simulink model "obstacleAvoidanceUsingOpticalFlow"  (R2021a)
settings: Solver=VariableStepAuto  StartTime=0.0  StopTime=30  RelTol=1e-3
PostLoadFcn:
  | %Add subfolders to path
  | addpath('virtualworld');
InitFcn:
  | startScript;
values from neighbouring files (symbols this model uses):
  angularVelocity = [0 0 -0.01]    [startScript.m]
  angularVelocityforLanding = [0 0 0.01]    [startScript.m]
  delta = 0.1    [startScript.m]
  dronestartlocation = [-1.5 0 4]    [startScript.m]
  finalHoverHeight = 0.8    [startScript.m]
  helipadLocation = [14 0.29 4]    [startScript.m]
  linearVelocity = [0.6 0.05 .2]    [startScript.m]
  switchingXLimit = 12.0    (= 12)    [startScript.m]
undefined symbols (not defined in the file or in its folder): gcbh, Horn, Rec, Schunck, SDTV, vrmfunc
libraries: vrlib x6, pid_lib x4, sharedtransform x2, visionconversions x1, visiontextngfix x1, visionanalysis x1
settings Model: Creator=91967  LastModifiedBy=mmordeka
settings SolverCC: AlgebraicLoopSolver=TrustRegion
settings DebuggingCC: SFMachineParentedDataDiag=warning

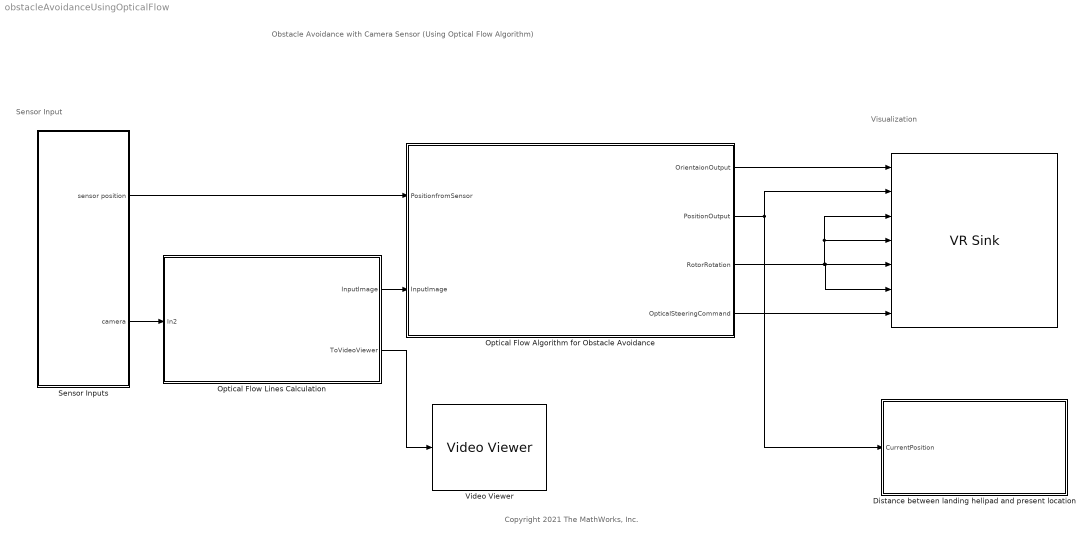
== system obstacleAvoidanceUsingOpticalFlow ==
  note: Sensor Input
  note: Copyright 2021 The MathWorks, Inc.
  note: Obstacle Avoidance with Camera Sensor
      | (Using Optical Flow Algorithm)
  note: Visualization
  "    " : vrlib/VR Sink  InstantiateOnLoad=on  SampleTime=0.04  ViewEnable=on  RemoteChange=off  RemoteView=off  FieldsWritten=UAV.rotation.4.1.1.double#UAV.translation.3.1.1.double#UAV_Body.Propeller_Mode_1.1.1.1.double#UAV_Body.Propeller_Mode_2.1.1.1.double#UAV_Body.Propeller_Mode_3.1.1.1.double#UAV_Body.Propeller_Mode_4.1.1.1.double#HUDText1.string.1.-1.1.char  WorldFileName=slv3.x3d  WorldDescription=Obstacle Avoidance with Camera Sensor (Using Optical Flow Algorithm)  AutoView=off  VideoDimensions=[]  AllowVariableSize=off
  " Distance between landing helipad and present location" : Subsystem
  " Optical Flow Algorithm for Obstacle Avoidance" : Subsystem
  Optical Flow Lines Calculation : Subsystem
  Sensor Inputs : Subsystem
  Video Viewer : VideoViewer  FigPos=[1242 576 441 340]  OpenAtMdlStart=off
  wires:
  " Optical Flow Algorithm for Obstacle Avoidance"/2(PositionOutput) -> " Distance between landing helipad and present location"/1(CurrentPosition), "    "/2
  Optical Flow Lines Calculation/1(InputImage) -> " Optical Flow Algorithm for Obstacle Avoidance"/2(InputImage)
  Optical Flow Lines Calculation/2(ToVideoViewer) -> Video Viewer/1
  Sensor Inputs/1(sensor position) -> " Optical Flow Algorithm for Obstacle Avoidance"/1(PositionfromSensor)
  Sensor Inputs/2(camera) -> Optical Flow Lines Calculation/1(In2)
  " Optical Flow Algorithm for Obstacle Avoidance"/1(OrientaionOutput) -> "    "/1
  " Optical Flow Algorithm for Obstacle Avoidance"/3(RotorRotation) -> "    "/4, "    "/3, "    "/6, "    "/5
  " Optical Flow Algorithm for Obstacle Avoidance"/4(OpticalSteeringCommand) -> "    "/7

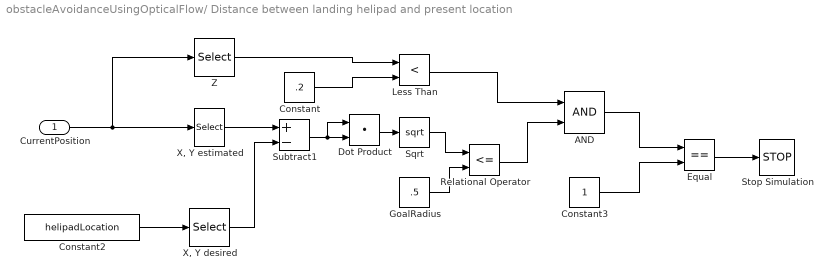
== system obstacleAvoidanceUsingOpticalFlow/ Distance between landing helipad and present location ==
  CurrentPosition : Inport
  AND : Logic  IconShape=distinctive  AllPortsSameDT=off  OutDataTypeStr=boolean
  Constant : Constant  Value=.2
  Constant2 : Constant  Value=helipadLocation
  Constant3 : Constant
  Dot Product : DotProduct  InputSameDT=on  OutDataTypeStr=Inherit: Inherit via internal rule
  Equal : RelationalOperator  Operator===  OutDataTypeStr=boolean  RndMeth=Simplest
  GoalRadius : Constant  Value=.5
  Less Than : RelationalOperator  Operator=<  OutDataTypeStr=boolean  RndMeth=Simplest
  Relational Operator : RelationalOperator  Operator=<=  OutDataTypeStr=boolean  RndMeth=Simplest
  Sqrt : Sqrt  SaturateOnIntegerOverflow=on
  Stop Simulation : Stop
  Subtract1 : Sum  Inputs=+-
  "X, Y desired" : Selector  InputPortWidth=3  IndexOptions=Index vector (dialog)  Indices=[1 3]  OutputSizes=1
  "X, Y estimated" : Selector  InputPortWidth=3  IndexOptions=Index vector (dialog)  Indices=[1 3]  OutputSizes=1
  Z : Selector  InputPortWidth=3  IndexOptions=Index vector (dialog)  Indices=[2]  OutputSizes=1
  wires:
  GoalRadius/1 -> Relational Operator/2
  Subtract1/1 -> Dot Product/1, Dot Product/2
  Dot Product/1 -> Sqrt/1
  Sqrt/1 -> Relational Operator/1
  "X, Y estimated"/1 -> Subtract1/1
  CurrentPosition/1 -> Z/1, "X, Y estimated"/1
  "X, Y desired"/1 -> Subtract1/2
  Constant3/1 -> Equal/2
  Equal/1 -> Stop Simulation/1
  Constant2/1 -> "X, Y desired"/1
  AND/1 -> Equal/1
  Relational Operator/1 -> AND/2
  Z/1 -> Less Than/1
  Constant/1 -> Less Than/2
  Less Than/1 -> AND/1

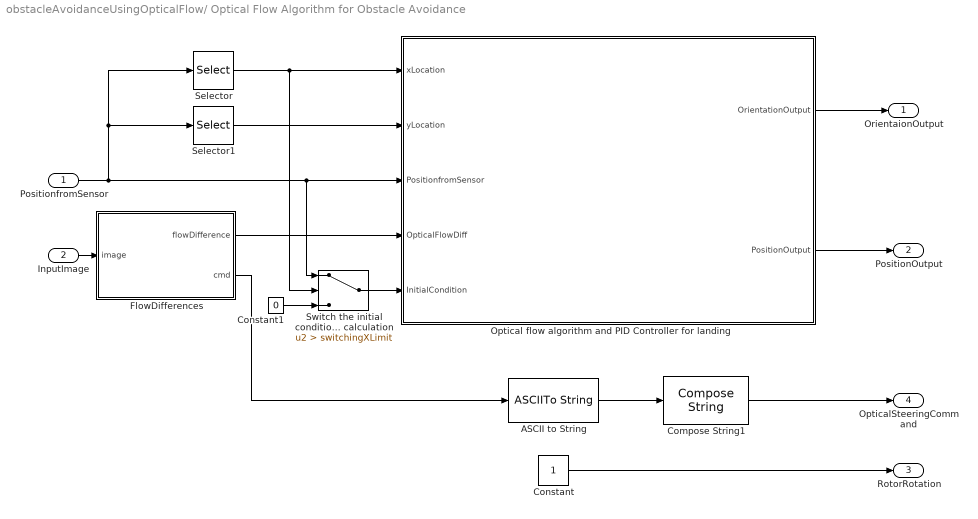
== system obstacleAvoidanceUsingOpticalFlow/ Optical Flow Algorithm for Obstacle Avoidance ==
  PositionfromSensor : Inport
  InputImage : Inport  Port=2
  ASCII to String : ASCIIToString
  Compose String1 : ComposeString  Format="\"%s\""
  Constant : Constant
  Constant1 : Constant  Value=0
  FlowDifferences : MATLAB Function  TreatAsAtomicUnit=on
  Optical flow algorithm and PID Controller for landing : Stateflow chart  TreatAsAtomicUnit=on
  Selector : Selector  InputPortWidth=3  IndexOptions=Index vector (dialog)  Indices=[1]  OutputSizes=1
  Selector1 : Selector  InputPortWidth=3  IndexOptions=Index vector (dialog)  Indices=[3]  OutputSizes=1
  Switch the initial condition for position calculation : Switch  Criteria=u2 > Threshold  Threshold=switchingXLimit
  OrientaionOutput : Outport
  PositionOutput : Outport  Port=2
  RotorRotation : Outport  Port=3
  OpticalSteeringCommand : Outport  Port=4
  wires:
  Optical flow algorithm and PID Controller for landing/2(PositionOutput) -> PositionOutput/1
  Optical flow algorithm and PID Controller for landing/1(OrientationOutput) -> OrientaionOutput/1
  PositionfromSensor/1 -> Selector/1, Selector1/1, Switch the initial condition for position calculation/1, Optical flow algorithm and PID Controller for landing/3(PositionfromSensor)
  Selector/1 -> Switch the initial condition for position calculation/2, Optical flow algorithm and PID Controller for landing/1(xLocation)
  InputImage/1 -> FlowDifferences/1(image)
  FlowDifferences/1(flowDifference) -> Optical flow algorithm and PID Controller for landing/4(OpticalFlowDiff)
  ASCII to String/1 -> Compose String1/1
  FlowDifferences/2(cmd) -> ASCII to String/1
  Compose String1/1 -> OpticalSteeringCommand/1
  Switch the initial condition for position calculation/1 -> Optical flow algorithm and PID Controller for landing/5(InitialCondition)
  Constant1/1 -> Switch the initial condition for position calculation/3
  Selector1/1 -> Optical flow algorithm and PID Controller for landing/2(yLocation)
  Constant/1 -> RotorRotation/1

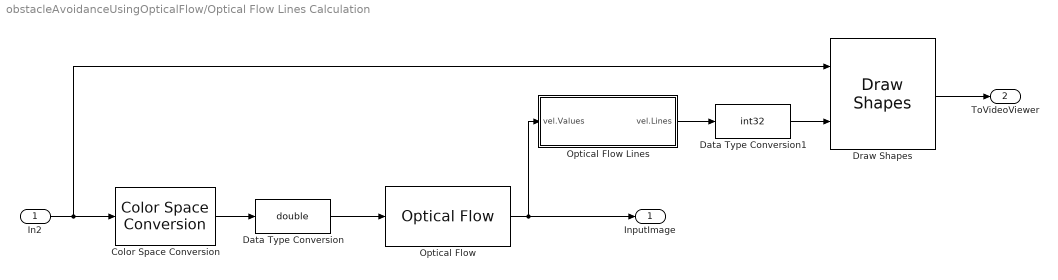
== system obstacleAvoidanceUsingOpticalFlow/Optical Flow Lines Calculation ==
  In2 : Inport
  Color Space Conversion : visionconversions/Color Space  Conversion  conversion=Obsolete  conversionActive=R'G'B' to intensity  wp_str=D65  rec=Rec. 601 (SDTV)  sys=1125/60/2:1  imagePorts=One multidimensional signal
  Data Type Conversion : DataTypeConversion  OutDataTypeStr=double
  Data Type Conversion1 : DataTypeConversion  OutDataTypeStr=int32
  Draw Shapes : visiontextngfix/Draw Shapes  shape=Lines  fill=off  lineWidth=1  fillClrSource=Specify via dialog  display=User-specified value  intensity=200  color=[255 255 0]  opacity=0.6  viewport=Entire image  antialiasing=off  inType=Obsolete  imagePorts=One multidimensional signal  roundingMode=Floor  overflowMode=off  memoryMode=Specify word length  memoryWordLength=16  prodOutputMode=Binary point scaling  prodOutputWordLength=32  prodOutputFracLength=14  memoryFracLength=15
  Optical Flow : visionanalysis/Optical Flow  method=Horn-Schunck  gradMethod=Difference filter [-1 1]  which2img=Current frame and N-th frame back  N=1  lambda=1  numInports=3  sigmaS=1.5  sigmaW=1  discardNormalFlow=off  outputCurrentImage=off  stop_criteria=When maximum number of iterations is reached  maxIter=10  maxAllowAbsDiff=eps  outVelForm=Magnitude-squared  eigTh=0.0039  roundingMode=Nearest  overflowMode=on  prodOutputMode=Binary point scaling  prodOutputWordLength=32  prodOutputFracLength=20  outputMode=Binary point scaling  outputWordLength=32  outputFracLength=20
      settings: SourceProductBaseCode=VP
  Optical Flow Lines : Subsystem  mask(Optical Flow Lines){scaleFactor=1}
      mask prompts: scaleFactor "Motion vector gain:"
      mask help: Generates the coordinate points of optical flow lines.
      mask Help: Generates the coordinate points of optical flow lines. Look under its mask to see the implementation details.
  InputImage : Outport
  ToVideoViewer : Outport  Port=2
  wires:
  Optical Flow Lines/1(vel.Lines) -> Data Type Conversion1/1
  Data Type Conversion1/1 -> Draw Shapes/2
  Optical Flow/1 -> InputImage/1, Optical Flow Lines/1(vel.Values)
  Draw Shapes/1 -> ToVideoViewer/1
  Data Type Conversion/1 -> Optical Flow/1
  In2/1 -> Draw Shapes/1, Color Space Conversion/1
  Color Space Conversion/1 -> Data Type Conversion/1

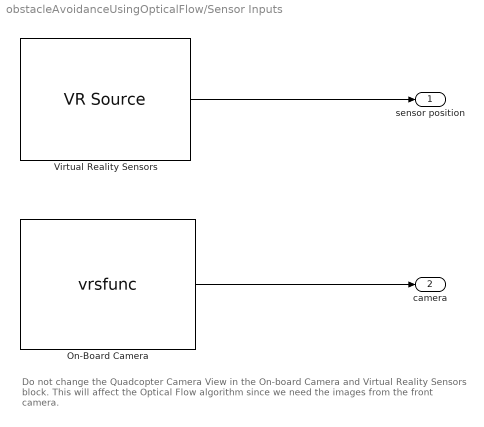
== system obstacleAvoidanceUsingOpticalFlow/Sensor Inputs ==
  note: Do not change the Quadcopter Camera View in the On-board Camera and Virtual Reality Sensors block. This will affect the Optical Flow algorithm since we need the images from the front camera.
  On-Board Camera : S-Function  InstantiateOnLoad=on  LoadFcn=vrmfunc('FnLoad', gcbh);  InitFcn=""  StartFcn=vrmfunc('FnSimStatus', gcbh, 'running')  StopFcn=vrmfunc('FnStop', gcbh)  FunctionName=vrsfunc  Parameters=SampleTime, VideoDimensions, false  SFunctionDeploymentMode=off  EnableBusSupport=off  mask(Virtual Reality Sink){SampleTime=0.04, ViewEnable=on, RemoteChange=off, RemoteView=off, FieldsWritten=, WorldFileName=slv3.x3d, WorldDescription=Obstacle avoidance using  Optical Flow Algorithm for UAV, AutoView=off, VideoDimensions=[320 480], AllowVariableSize=off, FigureProperties={'Position', 'Name', 'Viewpoint', 'CameraBound', 'CameraDirection', 'CameraPosition', 'CameraUpVector', 'ZoomFactor', 'Antialiasing', 'Headlight', 'Lighting', 'NavPanel', 'Sound', 'StatusBar', 'Stereo3D', 'Stereo3DCameraOffset', 'Stereo3DHIT', 'ToolBar', 'Textures', 'Transparency', 'Triad', 'Wireframe', 'NavZones', 'NavMode', 'NavSpeed', 'CaptureFileFormat', 'CaptureFileName', 'Record2DCompressMethod', 'Record2DCompressQuality', 'Record2D', 'Record2DFileName', 'Record2DFPS'; [5.8600000000000000e+02   6.0000000000000000e+01   4.8000000000000000e+02   3.2000000000000000e+02], 'UAV Competition Scene', 'Bird''s Eye', 'on', [0.0000000000000000e+00   0.0000000000000000e+00  -1.0000000000000000e+00], [0.0000000000000000e+00   0.0000000000000000e+00   0.0000000000000000e+00], [0.0000000000000000e+00   1.0000000000000000e+00   0.0000000000000000e+00], [1.0000000000000000e+00], 'on', 'on', 'on', 'none', 'on', 'off', 'off', [1.0000000149011612e-01], [0.0000000000000000e+00], 'off', 'on', 'on', 'none', 'off', 'off', 'fly', 'normal', 'tif', '%f_anim_%n.tif', 'auto', [7.5000000000000000e+01], 'off', '***video***', 'auto'}}
      mask prompts: SampleTime "Sample Time"; ViewEnable "View"; RemoteChange "Remote Change"; RemoteView "Remote View"; FieldsWritten "Fields Written"; WorldFileName "World File Name"; WorldDescription "World Description"; VideoDimensions "Video Dimensions"; AllowVariableSize "Allow Variable Size"; FigureProperties "Figure Properties"
      mask help: Controls the selected fields of a virtual world according to given inputs.
      mask init:
      | set_param(gcbh, 'MaskDisplay', vrmfunc('FnIcon'));
      settings: CopyFcn=vrmfunc('FnCopy', gcbh);  DeleteFcn=vrmfunc('FnDelete', gcbh);  PreSaveFcn=vrmfunc('FnPreSave', gcbh);  PauseFcn=vrmfunc('FnSimStatus', gcbh, 'paused');  ContinueFcn=vrmfunc('FnSimStatus', gcbh, 'running');  DestroyFcn=vrmfunc('FnDestroy', gcbh);  OpenFcn=vrmfunc('FnOpen', gcbh);  CloseFcn=vrmfunc('FnClose', gcbh);
      mask Help: helpview(vrmfunc('FnHelpTopic'), 'vr_vrtovideo');
      mask Display: image(imread('vrblockicon.png'));
  Virtual Reality Sensors : vrlib/VR Source  InstantiateOnLoad=on  SampleTime=0.04  ViewEnable=on  RemoteChange=off  RemoteView=off  FieldsRead=UAV.translation.1.3.1.double  WorldFileName=slv3.x3d  WorldDescription=UAV Competition Scene  AutoView=on  VideoDimensions=[]  AllowVariableSize=off  FigureProperties="{'Position', 'Name', 'Viewpoint', 'CameraBound', 'CameraDirection', 'CameraPosition', 'CameraUpVector', 'ZoomFactor', 'Antialiasing', 'Headlight', 'Lighting', 'NavPanel', 'Sound', 'StatusBar', 'Stereo3D', 'Stereo3DCameraOffset', 'Stereo3DHIT', 'ToolBar', 'Textures', 'Transparency', 'Triad', 'Wireframe', 'NavZones', 'NavMode', 'NavSpeed', 'CaptureFileFormat', 'CaptureFileName', 'Record2DCompressMethod', 'Record2DCompressQuality', 'Record2D', 'Record2DFileName', 'Record2DFPS'; [5.0000000000000000e+00   9.2000000000000000e+01   1.1190000000000000e+03   8.8800000000000000e+02], 'Obstacle avoidance using  Optical Flow Algorithm for UAV', 'View from the Top', 'on', [0.0000000000000000e+00   0.0000000000000000e+00  -1.0000000000000000e+00], [0.0000000000000000e+00   0.0000000000000000e+00   0.0000000000000000e+00], [0.0000000000000000e+00   1.0000000000000000e+00   0.0000000000000000e+00], [1.0000000000000000e+00], 'off', 'on', 'on', 'halfbar', 'on', 'on', 'off', [1.0000000149011612e-01], [0.0000000000000000e+00], 'on', 'on', 'on', 'none', 'off', 'off', 'fly', 'normal', 'tif', '%f_anim_%n.tif', 'auto', [7.5000000000000000e+01], 'off', '%f_anim_%n.avi', 'auto'}"
      settings: SourceProductBaseCode=SL
  sensor position : Outport
  camera : Outport  Port=2
  wires:
  On-Board Camera/1 -> camera/1
  Virtual Reality Sensors/1 -> sensor position/1

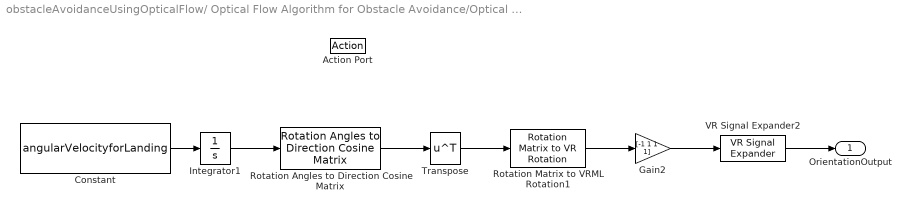
== system obstacleAvoidanceUsingOpticalFlow/ Optical Flow Algorithm for Obstacle Avoidance/Optical flow algorithm and PID Controller for landing/DroneOrientationEstimation.ControlAlgorithm_ ==
  Action Port : ActionPort
      settings: CopyFcn=Stateflow.SLINSF.SimulinkMan.removeBlockPreDeleteFcn  PreDeleteFcn=Stateflow.SLINSF.SimulinkMan.unsafePredeleteFcn
  Constant : Constant  Value=angularVelocityforLanding
  Gain2 : Gain  Gain=[-1 1 1 1]
  Integrator1 : Integrator
  Rotation Angles to Direction Cosine Matrix : sharedtransform/Rotation Angles to Direction Cosine Matrix  rotationOrder=YZX  aMode=aMode
      settings: SourceProductBaseCode=AE,PW,DR,MT,UV,VE
  Rotation Matrix to VRML Rotation1 : vrlib/Utilities/Rotation Matrix to VR Rotation  maxzero=1e-12
      settings: SourceProductBaseCode=SL
  Transpose : Math  Operator=transpose  SaturateOnIntegerOverflow=on
  VR Signal Expander2 : vrlib/VR Signal Expander  outwidth=4  outidx=[1 2 3 4]
  OrientationOutput : Outport
  wires:
  Rotation Matrix to VRML Rotation1/1 -> Gain2/1
  Constant/1 -> Integrator1/1
  Rotation Angles to Direction Cosine Matrix/1 -> Transpose/1
  Transpose/1 -> Rotation Matrix to VRML Rotation1/1
  VR Signal Expander2/1 -> OrientationOutput/1
  Integrator1/1 -> Rotation Angles to Direction Cosine Matrix/1
  Gain2/1 -> VR Signal Expander2/1

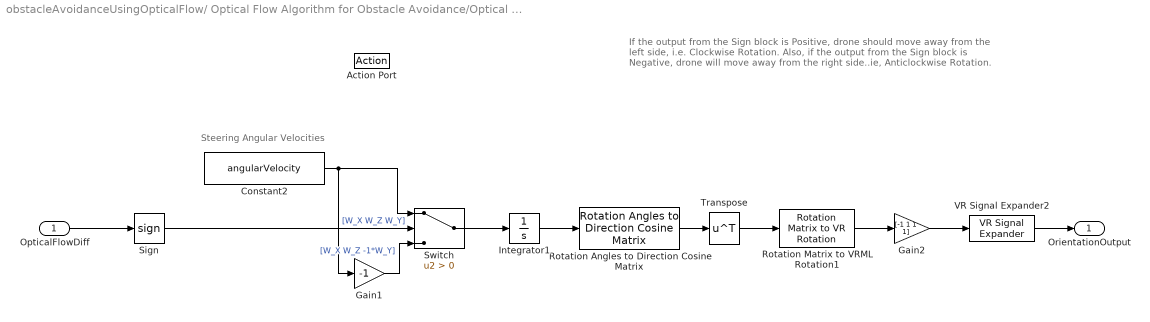
== system obstacleAvoidanceUsingOpticalFlow/ Optical Flow Algorithm for Obstacle Avoidance/Optical flow algorithm and PID Controller for landing/DroneOrientationEstimation.OpticalFlowAlgorithm_ ==
  note: If the output from the Sign block is Positive, drone should move away
      | from the left side, i.e. Clockwise Rotation. Also, if the output from the Sign
      |  block is Negative, drone will move away from the right side..ie,
      | Anticlockwise Rotation.
  note: Steering Angular Velocities
  OpticalFlowDiff : Inport
  Action Port : ActionPort
      settings: CopyFcn=Stateflow.SLINSF.SimulinkMan.removeBlockPreDeleteFcn  PreDeleteFcn=Stateflow.SLINSF.SimulinkMan.unsafePredeleteFcn
  Constant2 : Constant  Value=angularVelocity
  Gain1 : Gain  Gain=-1
  Gain2 : Gain  Gain=[-1 1 1 1]
  Integrator1 : Integrator
  Rotation Angles to Direction Cosine Matrix : sharedtransform/Rotation Angles to Direction Cosine Matrix  rotationOrder=YZX  aMode=aMode
      settings: SourceProductBaseCode=AE,PW,DR,MT,UV,VE
  Rotation Matrix to VRML Rotation1 : vrlib/Utilities/Rotation Matrix to VR Rotation  maxzero=1e-12
      settings: SourceProductBaseCode=SL
  Sign : Signum
  Switch : Switch  Criteria=u2 > Threshold
  Transpose : Math  Operator=transpose  SaturateOnIntegerOverflow=on
  VR Signal Expander2 : vrlib/VR Signal Expander  outwidth=4  outidx=[1 2 3 4]
  "OrientationOutput " : Outport
  wires:
  Transpose/1 -> Rotation Matrix to VRML Rotation1/1
  Integrator1/1 -> Rotation Angles to Direction Cosine Matrix/1
  VR Signal Expander2/1 -> "OrientationOutput "/1
  OpticalFlowDiff/1 -> Sign/1
  Rotation Angles to Direction Cosine Matrix/1 -> Transpose/1
  Rotation Matrix to VRML Rotation1/1 -> Gain2/1
  Switch/1 -> Integrator1/1
  Constant2/1 -> Switch/1, Gain1/1  "[W_X W_Z W_Y]"
  Sign/1 -> Switch/2
  Gain2/1 -> VR Signal Expander2/1
  Gain1/1 -> Switch/3  "[W_X W_Z -1*W_Y]"

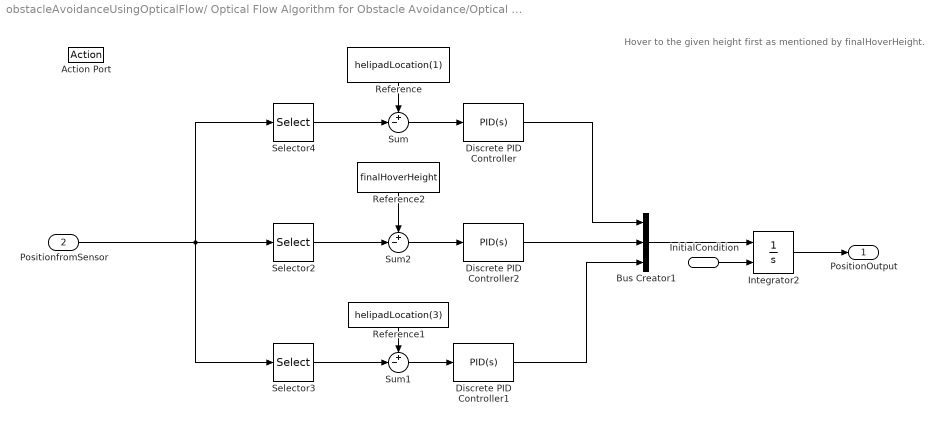
== system obstacleAvoidanceUsingOpticalFlow/ Optical Flow Algorithm for Obstacle Avoidance/Optical flow algorithm and PID Controller for landing/DronePositionEstimation.ControlAlgorithm_ ==
  note: Hover to the given height first as mentioned by finalHoverHeight.
  InitialCondition : Inport
  PositionfromSensor : Inport  Port=2
  Action Port : ActionPort
      settings: CopyFcn=Stateflow.SLINSF.SimulinkMan.removeBlockPreDeleteFcn  PreDeleteFcn=Stateflow.SLINSF.SimulinkMan.unsafePredeleteFcn
  Bus Creator1 : BusCreator  Inputs=3
  Discrete PID Controller : pid_lib/PID Controller  Controller=PID  Form=Parallel  TimeDomain=Continuous-time  UseExternalTs=off  SampleTime=-1  IntegratorMethod=Forward Euler  FilterMethod=Forward Euler  ControllerParametersSource=internal  P=10  I=0  D=0  UseFilter=on  N=100  TunerSelectOption=Transfer Function Based (PID Tuner App)  InitialConditionSource=internal  InitialConditionForIntegrator=0  InitialConditionForFilter=0  DifferentiatorICPrevScaledInput=0  ExternalReset=none  TrackingMode=off  Kt=1  LimitOutput=on  SatLimitsSource=internal  UpperSaturationLimit=1  LowerSaturationLimit=-1  LinearizeAsGain=off  AntiWindupMode=none  Kb=1  POutMin=[]  POutMax=[]  IOutMin=[]  IOutMax=[]  DOutMin=[]  DOutMax=[]  NOutMin=[]  NOutMax=[]  SumOutMin=[]  SumOutMax=[]  SaturationOutMin=[]  SaturationOutMax=[]  PParamMin=[]  PParamMax=[]  IParamMin=[]  IParamMax=[]  DParamMin=[]  DParamMax=[]  NParamMin=[]  NParamMax=[]  KbParamMin=[]  KbParamMax=[]  KtParamMin=[]  KtParamMax=[]  KbOutMin=[]  KbOutMax=[]  KtOutMin=[]  KtOutMax=[]  IntegratorOutMin=[]  IntegratorOutMax=[]  FilterOutMin=[]  FilterOutMax=[]  SumI1OutMin=[]  SumI1OutMax=[]  SumI2OutMin=[]  SumI2OutMax=[]  SumI3OutMin=[]  SumI3OutMax=[]  SumI4OutMin=[]  SumI4OutMax=[]  SumDOutMin=[]  SumDOutMax=[]  DifferentiatorOutMin=[]  DifferentiatorOutMax=[]  FilterDiffOutCoefMin=[]  FilterDiffOutCoefMax=[]  ReciprocalOutMin=[]  ReciprocalOutMax=[]  SumDenOutMin=[]  SumDenOutMax=[]  SumNumOutMin=[]  SumNumOutMax=[]  DivideOutMin=[]  DivideOutMax=[]  UdiffTsProdOutMin=[]  UdiffTsProdOutMax=[]  NTsProdOutMin=[]  NTsProdOutMax=[]  UintegralTsProdOutMin=[]  UintegralTsProdOutMax=[]  UngainTsProdOutMin=[]  UngainTsProdOutMax=[]  IntegratorContinuousStateAttributes=''  IntegratorStateMustResolveToSignalObject=off  IntegratorRTWStateStorageClass=Auto  FilterContinuousStateAttributes=''  FilterStateMustResolveToSignalObject=off  FilterRTWStateStorageClass=Auto  ParallelPVariant=InternalParameters  IdealPVariant=Disabled  IVariant=InternalParameters  DVariant=InternalParameters  IntegratorVariant=Continuous  SatVariant=Enabled  AWVariant=Passthrough  PCopyVariant=Disabled  TRVariant=Disabled  FdbkBlocksVariant=Forward  IdealPFdbkVariant=Disabled  SatFdbkVariant=Disabled  DerivativeFilterVariant=ContFilter  NVariant=InternalParameters  NCopyVariant=Disabled  FilterICVariant=InternalICsFilter  IntegratorICVariant=InternalICs  ExternalResetVariant=Disabled  TRSumVariant=Passthrough  SumFdbkVariant=Disabled  SumVariant=Sum_PID  TsampFilterVariant=InternalTs  TsampNgainVariant=Passthrough  TsampIntegralVariant=Passthrough  ExternalSaturationOutDataTypeStr=Inherit: Same as second input
  Discrete PID Controller1 : pid_lib/PID Controller  Controller=PID  Form=Parallel  TimeDomain=Continuous-time  UseExternalTs=off  SampleTime=-1  IntegratorMethod=Forward Euler  FilterMethod=Forward Euler  ControllerParametersSource=internal  P=10  I=0  D=0  UseFilter=on  N=100  TunerSelectOption=Transfer Function Based (PID Tuner App)  InitialConditionSource=internal  InitialConditionForIntegrator=0  InitialConditionForFilter=0  DifferentiatorICPrevScaledInput=0  ExternalReset=none  TrackingMode=off  Kt=1  LimitOutput=on  SatLimitsSource=internal  UpperSaturationLimit=1  LowerSaturationLimit=-1  LinearizeAsGain=off  AntiWindupMode=none  Kb=1  POutMin=[]  POutMax=[]  IOutMin=[]  IOutMax=[]  DOutMin=[]  DOutMax=[]  NOutMin=[]  NOutMax=[]  SumOutMin=[]  SumOutMax=[]  SaturationOutMin=[]  SaturationOutMax=[]  PParamMin=[]  PParamMax=[]  IParamMin=[]  IParamMax=[]  DParamMin=[]  DParamMax=[]  NParamMin=[]  NParamMax=[]  KbParamMin=[]  KbParamMax=[]  KtParamMin=[]  KtParamMax=[]  KbOutMin=[]  KbOutMax=[]  KtOutMin=[]  KtOutMax=[]  IntegratorOutMin=[]  IntegratorOutMax=[]  FilterOutMin=[]  FilterOutMax=[]  SumI1OutMin=[]  SumI1OutMax=[]  SumI2OutMin=[]  SumI2OutMax=[]  SumI3OutMin=[]  SumI3OutMax=[]  SumI4OutMin=[]  SumI4OutMax=[]  SumDOutMin=[]  SumDOutMax=[]  DifferentiatorOutMin=[]  DifferentiatorOutMax=[]  FilterDiffOutCoefMin=[]  FilterDiffOutCoefMax=[]  ReciprocalOutMin=[]  ReciprocalOutMax=[]  SumDenOutMin=[]  SumDenOutMax=[]  SumNumOutMin=[]  SumNumOutMax=[]  DivideOutMin=[]  DivideOutMax=[]  UdiffTsProdOutMin=[]  UdiffTsProdOutMax=[]  NTsProdOutMin=[]  NTsProdOutMax=[]  UintegralTsProdOutMin=[]  UintegralTsProdOutMax=[]  UngainTsProdOutMin=[]  UngainTsProdOutMax=[]  IntegratorContinuousStateAttributes=''  IntegratorStateMustResolveToSignalObject=off  IntegratorRTWStateStorageClass=Auto  FilterContinuousStateAttributes=''  FilterStateMustResolveToSignalObject=off  FilterRTWStateStorageClass=Auto  ParallelPVariant=InternalParameters  IdealPVariant=Disabled  IVariant=InternalParameters  DVariant=InternalParameters  IntegratorVariant=Continuous  SatVariant=Enabled  AWVariant=Passthrough  PCopyVariant=Disabled  TRVariant=Disabled  FdbkBlocksVariant=Forward  IdealPFdbkVariant=Disabled  SatFdbkVariant=Disabled  DerivativeFilterVariant=ContFilter  NVariant=InternalParameters  NCopyVariant=Disabled  FilterICVariant=InternalICsFilter  IntegratorICVariant=InternalICs  ExternalResetVariant=Disabled  TRSumVariant=Passthrough  SumFdbkVariant=Disabled  SumVariant=Sum_PID  TsampFilterVariant=InternalTs  TsampNgainVariant=Passthrough  TsampIntegralVariant=Passthrough  ExternalSaturationOutDataTypeStr=Inherit: Same as second input
  Discrete PID Controller2 : pid_lib/PID Controller  Controller=PID  Form=Parallel  TimeDomain=Continuous-time  UseExternalTs=off  SampleTime=-1  IntegratorMethod=Forward Euler  FilterMethod=Forward Euler  ControllerParametersSource=internal  P=1  I=0  D=0  UseFilter=on  N=100  TunerSelectOption=Transfer Function Based (PID Tuner App)  InitialConditionSource=internal  InitialConditionForIntegrator=0  InitialConditionForFilter=0  DifferentiatorICPrevScaledInput=0  ExternalReset=none  TrackingMode=off  Kt=1  LimitOutput=on  SatLimitsSource=internal  UpperSaturationLimit=1  LowerSaturationLimit=-1  LinearizeAsGain=off  AntiWindupMode=none  Kb=1  POutMin=[]  POutMax=[]  IOutMin=[]  IOutMax=[]  DOutMin=[]  DOutMax=[]  NOutMin=[]  NOutMax=[]  SumOutMin=[]  SumOutMax=[]  SaturationOutMin=[]  SaturationOutMax=[]  PParamMin=[]  PParamMax=[]  IParamMin=[]  IParamMax=[]  DParamMin=[]  DParamMax=[]  NParamMin=[]  NParamMax=[]  KbParamMin=[]  KbParamMax=[]  KtParamMin=[]  KtParamMax=[]  KbOutMin=[]  KbOutMax=[]  KtOutMin=[]  KtOutMax=[]  IntegratorOutMin=[]  IntegratorOutMax=[]  FilterOutMin=[]  FilterOutMax=[]  SumI1OutMin=[]  SumI1OutMax=[]  SumI2OutMin=[]  SumI2OutMax=[]  SumI3OutMin=[]  SumI3OutMax=[]  SumI4OutMin=[]  SumI4OutMax=[]  SumDOutMin=[]  SumDOutMax=[]  DifferentiatorOutMin=[]  DifferentiatorOutMax=[]  FilterDiffOutCoefMin=[]  FilterDiffOutCoefMax=[]  ReciprocalOutMin=[]  ReciprocalOutMax=[]  SumDenOutMin=[]  SumDenOutMax=[]  SumNumOutMin=[]  SumNumOutMax=[]  DivideOutMin=[]  DivideOutMax=[]  UdiffTsProdOutMin=[]  UdiffTsProdOutMax=[]  NTsProdOutMin=[]  NTsProdOutMax=[]  UintegralTsProdOutMin=[]  UintegralTsProdOutMax=[]  UngainTsProdOutMin=[]  UngainTsProdOutMax=[]  IntegratorContinuousStateAttributes=''  IntegratorStateMustResolveToSignalObject=off  IntegratorRTWStateStorageClass=Auto  FilterContinuousStateAttributes=''  FilterStateMustResolveToSignalObject=off  FilterRTWStateStorageClass=Auto  ParallelPVariant=InternalParameters  IdealPVariant=Disabled  IVariant=InternalParameters  DVariant=InternalParameters  IntegratorVariant=Continuous  SatVariant=Enabled  AWVariant=Passthrough  PCopyVariant=Disabled  TRVariant=Disabled  FdbkBlocksVariant=Forward  IdealPFdbkVariant=Disabled  SatFdbkVariant=Disabled  DerivativeFilterVariant=ContFilter  NVariant=InternalParameters  NCopyVariant=Disabled  FilterICVariant=InternalICsFilter  IntegratorICVariant=InternalICs  ExternalResetVariant=Disabled  TRSumVariant=Passthrough  SumFdbkVariant=Disabled  SumVariant=Sum_PID  TsampFilterVariant=InternalTs  TsampNgainVariant=Passthrough  TsampIntegralVariant=Passthrough  ExternalSaturationOutDataTypeStr=Inherit: Same as second input
  Integrator2 : Integrator  InitialConditionSource=external  InitialCondition=[9.1 0.5 6.2]  LimitOutput=on  UpperSaturationLimit=[40 10 20]  LowerSaturationLimit=[-5 0 -5]  ZeroCross=off
  Reference : Constant  Value=helipadLocation(1)
  Reference1 : Constant  Value=helipadLocation(3)
  Reference2 : Constant  Value=finalHoverHeight
  Selector2 : Selector  InputPortWidth=3  IndexOptions=Index vector (dialog)  Indices=[2]  OutputSizes=1
  Selector3 : Selector  InputPortWidth=3  IndexOptions=Index vector (dialog)  Indices=[3]  OutputSizes=1
  Selector4 : Selector  InputPortWidth=3  IndexOptions=Index vector (dialog)  Indices=[1]  OutputSizes=1
  Sum : Sum  Inputs=+-|
  Sum1 : Sum  Inputs=+-|
  Sum2 : Sum  Inputs=+-|
  PositionOutput : Outport
  wires:
  Discrete PID Controller2/1 -> Bus Creator1/2
  Sum2/1 -> Discrete PID Controller2/1
  Sum1/1 -> Discrete PID Controller1/1
  Reference1/1 -> Sum1/1
  Sum/1 -> Discrete PID Controller/1
  Reference2/1 -> Sum2/1
  Bus Creator1/1 -> Integrator2/1
  Discrete PID Controller1/1 -> Bus Creator1/3
  Selector2/1 -> Sum2/2
  Discrete PID Controller/1 -> Bus Creator1/1
  Reference/1 -> Sum/1
  Integrator2/1 -> PositionOutput/1
  Selector4/1 -> Sum/2
  PositionfromSensor/1 -> Selector4/1, Selector3/1, Selector2/1
  Selector3/1 -> Sum1/2
  InitialCondition/1 -> Integrator2/2

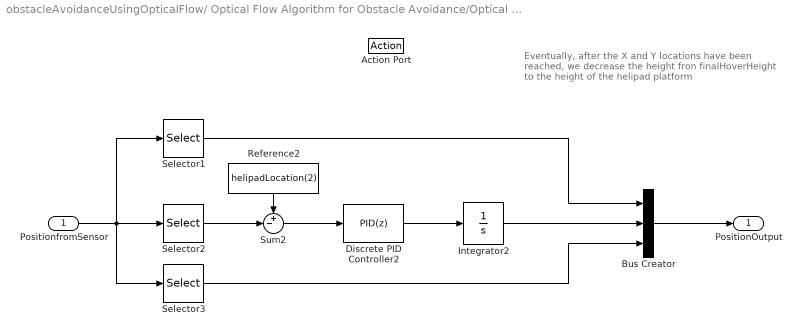
== system obstacleAvoidanceUsingOpticalFlow/ Optical Flow Algorithm for Obstacle Avoidance/Optical flow algorithm and PID Controller for landing/DronePositionEstimation.DroneLanding_ ==
  note: Eventually, after the X and Y locations have been reached, we decrease the height fron finalHoverHeight to the height of the helipad platform
  PositionfromSensor : Inport
  Action Port : ActionPort
      settings: CopyFcn=Stateflow.SLINSF.SimulinkMan.removeBlockPreDeleteFcn  PreDeleteFcn=Stateflow.SLINSF.SimulinkMan.unsafePredeleteFcn
  Bus Creator : BusCreator  Inputs=3
  Discrete PID Controller2 : pid_lib/PID Controller  Controller=PID  Form=Parallel  TimeDomain=Discrete-time  UseExternalTs=off  SampleTime=-1  IntegratorMethod=Forward Euler  FilterMethod=Forward Euler  ControllerParametersSource=internal  P=1  I=0  D=0  UseFilter=on  N=100  TunerSelectOption=Transfer Function Based (PID Tuner App)  InitialConditionSource=internal  InitialConditionForIntegrator=0  InitialConditionForFilter=0  DifferentiatorICPrevScaledInput=0  ExternalReset=none  TrackingMode=off  Kt=1  LimitOutput=on  SatLimitsSource=internal  UpperSaturationLimit=1  LowerSaturationLimit=-1  LinearizeAsGain=off  AntiWindupMode=none  Kb=1  POutMin=[]  POutMax=[]  IOutMin=[]  IOutMax=[]  DOutMin=[]  DOutMax=[]  NOutMin=[]  NOutMax=[]  SumOutMin=[]  SumOutMax=[]  SaturationOutMin=[]  SaturationOutMax=[]  PParamMin=[]  PParamMax=[]  IParamMin=[]  IParamMax=[]  DParamMin=[]  DParamMax=[]  NParamMin=[]  NParamMax=[]  KbParamMin=[]  KbParamMax=[]  KtParamMin=[]  KtParamMax=[]  KbOutMin=[]  KbOutMax=[]  KtOutMin=[]  KtOutMax=[]  IntegratorOutMin=[]  IntegratorOutMax=[]  FilterOutMin=[]  FilterOutMax=[]  SumI1OutMin=[]  SumI1OutMax=[]  SumI2OutMin=[]  SumI2OutMax=[]  SumI3OutMin=[]  SumI3OutMax=[]  SumI4OutMin=[]  SumI4OutMax=[]  SumDOutMin=[]  SumDOutMax=[]  DifferentiatorOutMin=[]  DifferentiatorOutMax=[]  FilterDiffOutCoefMin=[]  FilterDiffOutCoefMax=[]  ReciprocalOutMin=[]  ReciprocalOutMax=[]  SumDenOutMin=[]  SumDenOutMax=[]  SumNumOutMin=[]  SumNumOutMax=[]  DivideOutMin=[]  DivideOutMax=[]  UdiffTsProdOutMin=[]  UdiffTsProdOutMax=[]  NTsProdOutMin=[]  NTsProdOutMax=[]  UintegralTsProdOutMin=[]  UintegralTsProdOutMax=[]  UngainTsProdOutMin=[]  UngainTsProdOutMax=[]  IntegratorContinuousStateAttributes=''  IntegratorStateMustResolveToSignalObject=off  IntegratorRTWStateStorageClass=Auto  FilterContinuousStateAttributes=''  FilterStateMustResolveToSignalObject=off  FilterRTWStateStorageClass=Auto  ParallelPVariant=InternalParameters  IdealPVariant=Disabled  IVariant=InternalParameters  DVariant=InternalParameters  IntegratorVariant=Discrete  SatVariant=Enabled  AWVariant=Passthrough  PCopyVariant=Disabled  TRVariant=Disabled  FdbkBlocksVariant=Forward  IdealPFdbkVariant=Disabled  SatFdbkVariant=Disabled  DerivativeFilterVariant=ForwardEulerFilter  NVariant=InternalParameters  NCopyVariant=Disabled  FilterICVariant=InternalICsFilter  IntegratorICVariant=InternalICs  ExternalResetVariant=Disabled  TRSumVariant=Passthrough  SumFdbkVariant=Disabled  SumVariant=Sum_PID  TsampFilterVariant=InternalTs  TsampNgainVariant=Passthrough  TsampIntegralVariant=Passthrough  ExternalSaturationOutDataTypeStr=Inherit: Same as second input
  Integrator2 : Integrator  InitialCondition=finalHoverHeight  UpperSaturationLimit=[40 10 20]  LowerSaturationLimit=[-5 0 -5]  ZeroCross=off
  Reference2 : Constant  Value=helipadLocation(2)
  Selector1 : Selector  InputPortWidth=3  IndexOptions=Index vector (dialog)  Indices=[1]  OutputSizes=1
  Selector2 : Selector  InputPortWidth=3  IndexOptions=Index vector (dialog)  Indices=[2]  OutputSizes=1
  Selector3 : Selector  InputPortWidth=3  IndexOptions=Index vector (dialog)  Indices=[3]  OutputSizes=1
  Sum2 : Sum  Inputs=+-|
  PositionOutput : Outport
  wires:
  PositionfromSensor/1 -> Selector3/1, Selector1/1, Selector2/1
  Reference2/1 -> Sum2/1
  Selector2/1 -> Sum2/2
  Sum2/1 -> Discrete PID Controller2/1
  Discrete PID Controller2/1 -> Integrator2/1
  Selector1/1 -> Bus Creator/1
  Integrator2/1 -> Bus Creator/2
  Selector3/1 -> Bus Creator/3
  Bus Creator/1 -> PositionOutput/1

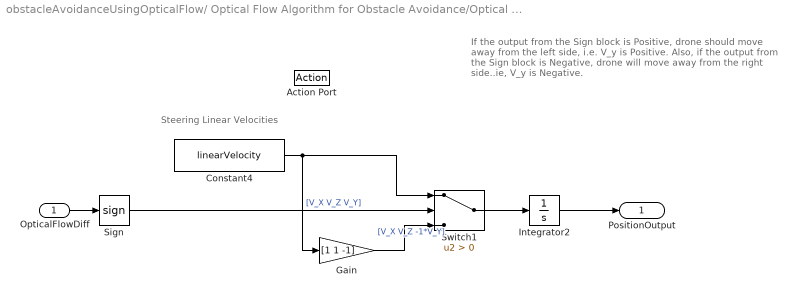
== system obstacleAvoidanceUsingOpticalFlow/ Optical Flow Algorithm for Obstacle Avoidance/Optical flow algorithm and PID Controller for landing/DronePositionEstimation.OpticalFlowAlgorithm_ ==
  note: If the output from the Sign block is Positive, drone should move away from the left side, i.e. V_y is Positive. Also, if the output from the Sign block is Negative, drone will move away from the right side..ie, V_y is Negative.
  note: Steering Linear Velocities
  OpticalFlowDiff : Inport
  Action Port : ActionPort
      settings: CopyFcn=Stateflow.SLINSF.SimulinkMan.removeBlockPreDeleteFcn  PreDeleteFcn=Stateflow.SLINSF.SimulinkMan.unsafePredeleteFcn
  Constant4 : Constant  Value=linearVelocity
  Gain : Gain  Gain=[1 1 -1]
  Integrator2 : Integrator  InitialCondition=dronestartlocation
  Sign : Signum
  Switch1 : Switch  Criteria=u2 > Threshold
  PositionOutput : Outport
  wires:
  Integrator2/1 -> PositionOutput/1
  OpticalFlowDiff/1 -> Sign/1
  Gain/1 -> Switch1/3  "[V_X V_Z -1*V_Y]"
  Sign/1 -> Switch1/2
  Constant4/1 -> Switch1/1, Gain/1  "[V_X V_Z V_Y]"
  Switch1/1 -> Integrator2/1

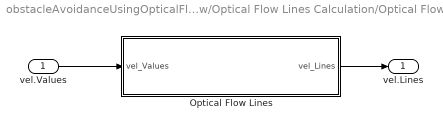
== system obstacleAvoidanceUsingOpticalFlow/Optical Flow Lines Calculation/Optical Flow Lines ==
  vel.Values : Inport
  Optical Flow Lines : MATLAB Function  TreatAsAtomicUnit=on
  vel.Lines : Outport
  wires:
  Optical Flow Lines/1(vel_Lines) -> vel.Lines/1
  vel.Values/1 -> Optical Flow Lines/1(vel_Values)

== stateflow chart obstacleAvoidanceUsingOpticalFlow/ Optical Flow Algorithm for Obstacle Avoidance/Optical flow algorithm and PID Controller for landing ==
  settings: updateMethod=CONTINUOUS
  state DronePositionEstimation [parallel]
    settings: executionOrder=1
    note: Controller for position is divided into three states:
        | Navigate left right based on optical flow lines
        | 2. Navigate the drone to hover over helipadLocation using PID controller
        | 3. Landing on the helipad from the height the drone was hovering at
    state OpticalFlowAlgorithm_
    state DroneLanding_
    state ControlAlgorithm_
    (default) -> DronePositionEstimation.OpticalFlowAlgorithm_
    DronePositionEstimation.OpticalFlowAlgorithm_ -> DronePositionEstimation.ControlAlgorithm_ : [xLocation>switchingXLimit]
    DronePositionEstimation.ControlAlgorithm_ -> (junction 41) [order 1] : [abs(yLocation-helipadLocation(3)) <= delta...
        | && abs(xLocation-helipadLocation(1)) <= delta]
    DronePositionEstimation.ControlAlgorithm_ -> DronePositionEstimation.OpticalFlowAlgorithm_ [order 2] : [xLocation<switchingXLimit]
    (junction 41) -> DroneLanding_ : after(1,sec)
    DroneLanding_ -> DronePositionEstimation.ControlAlgorithm_ : [xLocation<switchingXLimit]
  state DroneOrientationEstimation [parallel]
    settings: executionOrder=2
    note: Controller for orientation is divided into two parts:
        | Navigate left right based on optical flow lines
        | Constant angular velocity to move to helipadLocation
    state OpticalFlowAlgorithm_
    state ControlAlgorithm_
    (default) -> DroneOrientationEstimation.OpticalFlowAlgorithm_
    DroneOrientationEstimation.OpticalFlowAlgorithm_ -> DroneOrientationEstimation.ControlAlgorithm_ : [xLocation>switchingXLimit]
    DroneOrientationEstimation.ControlAlgorithm_ -> DroneOrientationEstimation.OpticalFlowAlgorithm_ : [xLocation<switchingXLimit]
  data: sf_internal_action_state_placeholder_data local double size=1 =0; sf_internal_action_state_placeholder_data local double size=1 =0; sf_internal_action_state_placeholder_data local double size=1 =0; sf_internal_action_state_placeholder_data local double size=1 =0; sf_internal_action_state_placeholder_data local double size=1 =0; OrientationOutput output; xLocation input; yLocation input; PositionfromSensor input; OpticalFlowDiff input; PositionOutput output; helipadLocation parameter; InitialCondition input; switchingXLimit local double; delta local

== matlab function obstacleAvoidanceUsingOpticalFlow/Optical Flow Lines Calculation/Optical Flow Lines/Optical Flow Lines ==
  data: vel_Values input; vel_Lines output; scaleFactor parameter size=1
function vel_Lines=OpticalFlowLines(vel_Values, scaleFactor) 

% Generates the coordinate points of optical flow lines

persistent first_time;
persistent X;
persistent Y;
persistent RV;
persistent CV;
if isempty(first_time)
    first_time     = 1;
    %% user may change the following three parameters
    borderOffset   = 5;
    decimFactorRow = 5;
    decimFactorCol = 5;    
    %%
    [R C] = size(vel_Values);
    RV = borderOffset:decimFactorRow:(R-borderOffset);   
    CV = borderOffset:decimFactorCol:(C-borderOffset);
    [Y X] = meshgrid(CV,RV);
end

tmp = vel_Values(RV,CV);
tmp = tmp.*scaleFactor;
vel_Lines = [Y(:), X(:), Y(:)+real(tmp(:)), X(:)+imag(tmp(:))];

== matlab function obstacleAvoidanceUsingOpticalFlow/ Optical Flow Algorithm for Obstacle Avoidance/FlowDifferences ==
  data: flowDifference output; cmd output; image input
function [flowDifference,cmd] = calculatethedifference(image)

% Image Preprocessing
image = flip(image, 1);

% Image Width
width = size(image,2);

% Calculate optical flow on right-half and the left-half of the image
VLeftFlow = image(:, 1:width/2); 
VRightFlow = image(:, width/2:width);

% Sum to get the total Optical Flow on the right-half and on left-half
vleftflow = sum(VLeftFlow(:));
vrightflow = sum(VRightFlow(:));

% Find the difference if the flow between the two halves
flowDifference = (vleftflow - vrightflow);

% Steer in the direction that has less optical flow which implies less 
% obstacles
if flowDifference>0
    cmd=uint8('Steering to Right');
else
    cmd=uint8('Steering to Left ');
end
